simulink library "BlockLib"  (R2014b)
settings: Solver=ode45  StartTime=0.0  StopTime=10.0  RelTol=1e-3
libraries: BlockLib x3, dspsrcs4 x1
settings Model: Creator=kunalmenda  LastModifiedBy=kunalmenda

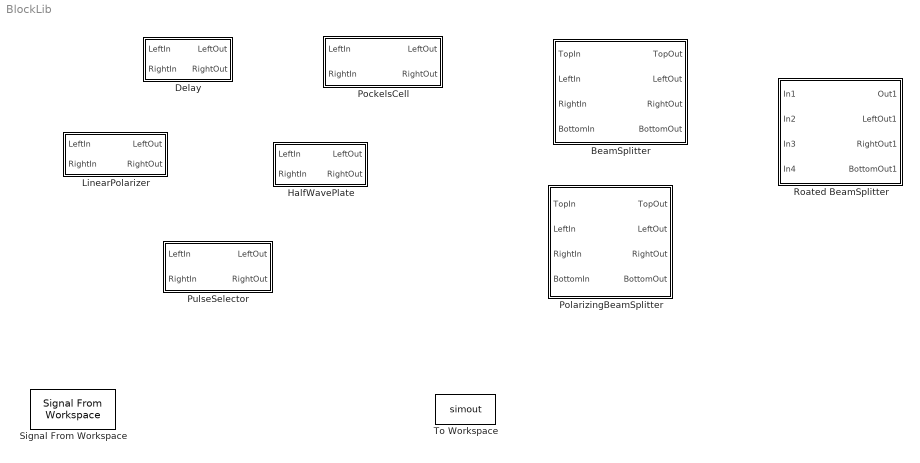
== system BlockLib ==
  BeamSplitter : Subsystem  mask{Transmittance=0.50, Reflectance=0.50, Ghost=0.01, BackReflectance=0.001}
      mask prompts: BackReflectance "Back Reflectance"
      mask TypeOptions Transmittance: BeamSplitter/Transmittance
      mask TypeOptions Reflectance: BeamSplitter/Reflectance
      mask TypeOptions Ghost: BeamSplitter/Ghost
      mask TypeOptions BackReflectance: BeamSplitter/BackReflectance
      mask Display:
      | image('BeamSplitter.jpg')
      | 
      | port_label('input',1,'TopIn');
      | port_label('input',2,'LeftIn');
      | port_label('input',3,'RightIn');
      | port_label('input',4,'BottomIn');
      | port_label('output',1,'TopOut');
      | port_label('output',2,'LeftOut');
      | port_label('output',3,'RightOut');
      | port_label('output',4,'BottomOut');
  Delay : Subsystem  mask{DelayAmt=10e-9}
      mask prompts: DelayAmt "Delay Amout"
      mask TypeOptions DelayAmt: Delay/DelayAmt
  HalfWavePlate : Subsystem  mask{Psi=pi/4, Transmittence=1}
      mask TypeOptions Psi: HalfWavePlate/Psi
      mask TypeOptions Transmittence: HalfWavePlate/Transmittence
  LinearPolarizer : Subsystem  mask{Psi=pi/4, Transmittence=0.81, ExtinctionRatio=200000000}
      mask TypeOptions Psi: LinearPolarizer/Psi
      mask TypeOptions Transmittence: LinearPolarizer/Transmittence
      mask TypeOptions ExtinctionRatio: LinearPolarizer/ExtinctionRatio
  PockelsCell : Subsystem  mask{PCTimings=[-1,1,38,40,103,105,168,170,220,274]*1e-9, ControlPowers=[0.5000, 1.0000,1.0000, 1.0000, 0.5000], Psi=pi/4}
      mask prompts: PCTimings "PC Timings"; ControlPowers "Control Powers"
      mask TypeOptions PCTimings: PockelsCell/PCTimings
      mask TypeOptions ControlPowers: PockelsCell/ControlPowers
      mask TypeOptions Psi: PockelsCell/Psi
  PolarizingBeamSplitter : Subsystem  mask{Psi=pi/2, Transmittance=0.50, Reflectance=0.50, Ghost=0.01, BackReflectance=0.001}
      mask prompts: BackReflectance "Back Reflectance"
      mask TypeOptions Psi: PolarizingBeamSplitter/Psi
      mask TypeOptions Transmittance: PolarizingBeamSplitter/Transmittance
      mask TypeOptions Reflectance: PolarizingBeamSplitter/Reflectance
      mask TypeOptions Ghost: PolarizingBeamSplitter/Ghost
      mask TypeOptions BackReflectance: PolarizingBeamSplitter/BackReflectance
      mask Display:
      | image('PolBeamSplitter.jpg')
      | 
      | port_label('input',1,'TopIn');
      | port_label('input',2,'LeftIn');
      | port_label('input',3,'RightIn');
      | port_label('input',4,'BottomIn');
      | port_label('output',1,'TopOut');
      | port_label('output',2,'LeftOut');
      | port_label('output',3,'RightOut');
      | port_label('output',4,'BottomOut');
  PulseSelector : Subsystem  mask{PCTimings=[-1,1,38,40,103,105,168,170,220,274]*1e-9, ControlPowers=[0.5000, 1.0000,1.0000, 1.0000, 0.5000]}
      mask prompts: PCTimings "PC Timings"; ControlPowers "Control Powers"
      mask TypeOptions PCTimings: PockelsCell/PCTimings
      mask TypeOptions ControlPowers: PockelsCell/ControlPowers
  Roated BeamSplitter : Subsystem  mask{Transmittance=0, Reflectance=0, Ghost=0, BackReflectance=0}
      mask TypeOptions Transmittance:
      | Level-2 MATLAB
      | S-Function/Transmittance
      mask TypeOptions Reflectance:
      | Level-2 MATLAB
      | S-Function/Reflectance
      mask TypeOptions Ghost:
      | Level-2 MATLAB
      | S-Function/Ghost
      mask TypeOptions BackReflectance:
      | Level-2 MATLAB
      | S-Function/BackReflectance
      mask Display:
      | image('BeamSplitterRot.jpeg')
      | 
      | port_label('input',1,'TopIn');
      | port_label('input',2,'LeftIn');
      | port_label('input',3,'RightIn');
      | port_label('input',4,'BottomIn');
      | port_label('output',1,'TopOut');
      | port_label('output',2,'LeftOut');
      | port_label('output',3,'RightOut');
      | port_label('output',4,'BottomOut');
  Signal From Workspace : dspsrcs4/Signal From Workspace  X=inputsignal  Ts=1  nsamps=1  OutputAfterFinalValue=Setting to zero  ignoreOrWarnInputAndFrameLengths=off
  To Workspace : ToWorkspace  VariableName=simout  SaveFormat=Timeseries  SampleTime=-1

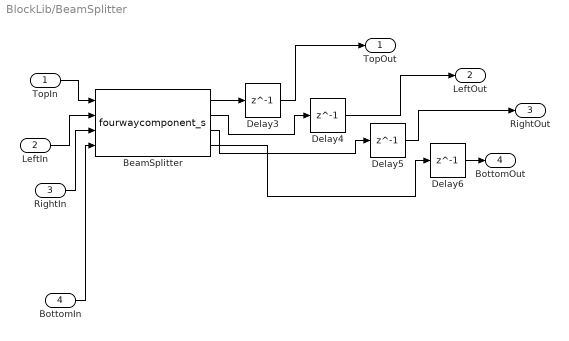
== system BlockLib/BeamSplitter ==
  TopIn : Inport
  LeftIn : Inport  Port=2
  RightIn : Inport  Port=3
  BottomIn : Inport  Port=4
  BeamSplitter : M-S-Function  FunctionName=fourwaycomponent_s  Parameters='BeamSplitter',Params  mask{Transmittance=Transmittance, Reflectance=Reflectance, Ghost=Ghost, BackReflectance=BackReflectance}
      mask prompts: BackReflectance "Back Reflectance"
      mask init:
      | Params.Transmittance = Transmittance;
      | Params.Reflectance = Reflectance;
      | Params.Ghost = Ghost;
      | Params.BackReflectance = BackReflectance;
      mask Display:
      | port_label('input',1,'TopIn');
      | port_label('input',2,'LeftIn');
      | port_label('input',3,'RightIn');
      | port_label('input',4,'BottomIn');
      | port_label('output',1,'TopOut');
      | port_label('output',2,'LeftOut');
      | port_label('output',3,'RightOut');
      | port_label('output',4,'BottomOut');
  Delay{3..6} (4 alike) : Delay  DelayLength=1  InitialCondition=0
  TopOut : Outport
  LeftOut : Outport  Port=2
  RightOut : Outport  Port=3
  BottomOut : Outport  Port=4
  wires:
  BeamSplitter/2 -> Delay4/1
  RightIn/1 -> BeamSplitter/3
  LeftIn/1 -> BeamSplitter/2
  Delay3/1 -> TopOut/1
  Delay4/1 -> LeftOut/1
  Delay6/1 -> BottomOut/1
  TopIn/1 -> BeamSplitter/1
  BottomIn/1 -> BeamSplitter/4
  BeamSplitter/1 -> Delay3/1
  BeamSplitter/3 -> Delay5/1
  Delay5/1 -> RightOut/1
  BeamSplitter/4 -> Delay6/1

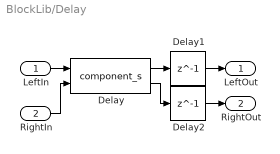
== system BlockLib/Delay ==
  LeftIn : Inport
  RightIn : Inport  Port=2
  Delay : M-S-Function  FunctionName=component_s  Parameters='Delay',Params  mask{DelayAmt=DelayAmt}
      mask prompts: DelayAmt "Delay Amout"
      mask init:
      | Params.DelayAmt = DelayAmt;
      mask Display:
      | port_label('input',1,'LeftIn');
      | port_label('input',2,'RightIn');
      | port_label('output',1,'LeftOut');
      | port_label('output',2,'RightOut');
  Delay1 : Delay  DelayLength=1  InitialCondition=0
  Delay2 : Delay  DelayLength=1  InitialCondition=0
  LeftOut : Outport
  RightOut : Outport  Port=2
  wires:
  Delay/1 -> Delay1/1
  Delay/2 -> Delay2/1
  LeftIn/1 -> Delay/1
  RightIn/1 -> Delay/2
  Delay1/1 -> LeftOut/1
  Delay2/1 -> RightOut/1

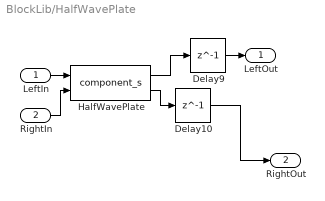
== system BlockLib/HalfWavePlate ==
  LeftIn : Inport
  RightIn : Inport  Port=2
  Delay10 : Delay  DelayLength=1  InitialCondition=0
  Delay9 : Delay  DelayLength=1  InitialCondition=0
  HalfWavePlate : M-S-Function  FunctionName=component_s  Parameters='HalfWavePlate',Params  mask{Psi=Psi, Transmittence=Transmittence}
      mask init:
      | Params.Psi = Psi;
      | Params.Transmittence = Transmittence;
      mask Display:
      | port_label('input',1,'LeftIn');
      | port_label('input',2,'RightIn');
      | port_label('output',1,'LeftOut');
      | port_label('output',2,'RightOut');
  LeftOut : Outport
  RightOut : Outport  Port=2
  wires:
  HalfWavePlate/1 -> Delay9/1
  Delay9/1 -> LeftOut/1
  LeftIn/1 -> HalfWavePlate/1
  RightIn/1 -> HalfWavePlate/2
  HalfWavePlate/2 -> Delay10/1
  Delay10/1 -> RightOut/1

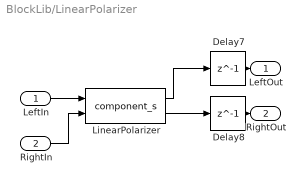
== system BlockLib/LinearPolarizer ==
  LeftIn : Inport
  RightIn : Inport  Port=2
  Delay7 : Delay  DelayLength=1  InitialCondition=0
  Delay8 : Delay  DelayLength=1  InitialCondition=0
  LinearPolarizer : M-S-Function  FunctionName=component_s  Parameters='LinearPolarizer',Params  mask{Psi=Psi, Transmittence=Transmittence, ExtinctionRatio=ExtinctionRatio}
      mask init:
      | Params.Psi = Psi;
      | Params.Transmittence = Transmittence;
      | Params.ExtinctionRatio = ExtinctionRatio;
      mask Display:
      | port_label('input',1,'LeftIn');
      | port_label('input',2,'RightIn');
      | port_label('output',1,'LeftOut');
      | port_label('output',2,'RightOut');
  LeftOut : Outport
  RightOut : Outport  Port=2
  wires:
  Delay8/1 -> RightOut/1
  RightIn/1 -> LinearPolarizer/2
  Delay7/1 -> LeftOut/1
  LeftIn/1 -> LinearPolarizer/1
  LinearPolarizer/1 -> Delay7/1
  LinearPolarizer/2 -> Delay8/1

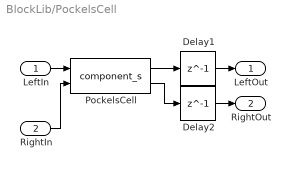
== system BlockLib/PockelsCell ==
  LeftIn : Inport
  RightIn : Inport  Port=2
  Delay1 : Delay  DelayLength=1  InitialCondition=0
  Delay2 : Delay  DelayLength=1  InitialCondition=0
  PockelsCell : M-S-Function  FunctionName=component_s  Parameters='PockelsCell',Params  mask{PCTimings=PCTimings, ControlPowers=ControlPowers, Psi=Psi}
      mask prompts: PCTimings "PC Timings"; ControlPowers "Control Powers"
      mask init:
      | Params.PCTimings = PCTimings;
      | Params.ControlPowers = ControlPowers;
      | Params.Psi = Psi;
      mask Display:
      | port_label('input',1,'LeftIn');
      | port_label('input',2,'RightIn');
      | port_label('output',1,'LeftOut');
      | port_label('output',2,'RightOut');
  LeftOut : Outport
  RightOut : Outport  Port=2
  wires:
  RightIn/1 -> PockelsCell/2
  PockelsCell/1 -> Delay1/1
  LeftIn/1 -> PockelsCell/1
  PockelsCell/2 -> Delay2/1
  Delay2/1 -> RightOut/1
  Delay1/1 -> LeftOut/1

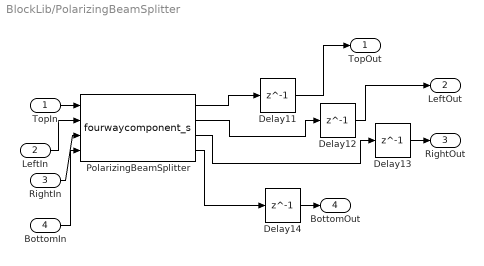
== system BlockLib/PolarizingBeamSplitter ==
  TopIn : Inport
  LeftIn : Inport  Port=2
  RightIn : Inport  Port=3
  BottomIn : Inport  Port=4
  Delay{11..14} (4 alike) : Delay  DelayLength=1  InitialCondition=0
  PolarizingBeamSplitter : M-S-Function  FunctionName=fourwaycomponent_s  Parameters='PolarizingBeamSplitter',Params  mask{Psi=Psi, Transmittance=Transmittance, Reflectance=Reflectance, Ghost=Ghost, BackReflectance=BackReflectance}
      mask prompts: BackReflectance "Back Reflectance"
      mask init:
      | Params.Psi = Psi;
      | Params.Transmittance = Transmittance;
      | Params.Reflectance = Reflectance;
      | Params.Ghost = Ghost;
      | Params.BackReflectance = BackReflectance;
      mask Display:
      | port_label('input',1,'TopIn');
      | port_label('input',2,'LeftIn');
      | port_label('input',3,'RightIn');
      | port_label('input',4,'BottomIn');
      | port_label('output',1,'TopOut');
      | port_label('output',2,'LeftOut');
      | port_label('output',3,'RightOut');
      | port_label('output',4,'BottomOut');
  TopOut : Outport
  LeftOut : Outport  Port=2
  RightOut : Outport  Port=3
  BottomOut : Outport  Port=4
  wires:
  RightIn/1 -> PolarizingBeamSplitter/3
  TopIn/1 -> PolarizingBeamSplitter/1
  Delay13/1 -> RightOut/1
  LeftIn/1 -> PolarizingBeamSplitter/2
  BottomIn/1 -> PolarizingBeamSplitter/4
  Delay11/1 -> TopOut/1
  Delay14/1 -> BottomOut/1
  Delay12/1 -> LeftOut/1
  PolarizingBeamSplitter/2 -> Delay12/1
  PolarizingBeamSplitter/1 -> Delay11/1
  PolarizingBeamSplitter/3 -> Delay13/1
  PolarizingBeamSplitter/4 -> Delay14/1

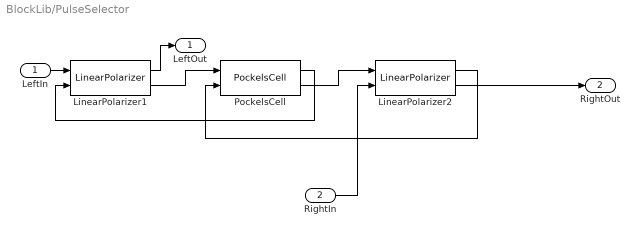
== system BlockLib/PulseSelector ==
  LeftIn : Inport
  RightIn : Inport  Port=2
  LinearPolarizer1 : BlockLib/LinearPolarizer  Psi=0  Transmittence=0.81  ExtinctionRatio=200000000
  LinearPolarizer2 : BlockLib/LinearPolarizer  Psi=pi/2  Transmittence=0.81  ExtinctionRatio=200000000
  PockelsCell : BlockLib/PockelsCell  PCTimings=PCTimings  ControlPowers=ControlPowers  Psi=pi/4
  LeftOut : Outport
  RightOut : Outport  Port=2
  wires:
  LeftIn/1 -> LinearPolarizer1/1
  LinearPolarizer1/2 -> PockelsCell/1
  PockelsCell/2 -> LinearPolarizer2/1
  RightIn/1 -> LinearPolarizer2/2
  LinearPolarizer2/1 -> PockelsCell/2
  PockelsCell/1 -> LinearPolarizer1/2
  LinearPolarizer1/1 -> LeftOut/1
  LinearPolarizer2/2 -> RightOut/1

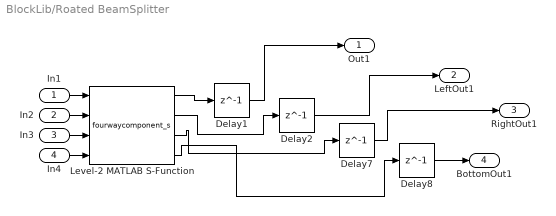
== system BlockLib/Roated BeamSplitter ==
  In1 : Inport
  In2 : Inport  Port=2
  In3 : Inport  Port=3
  In4 : Inport  Port=4
  Delay{1..2,7..8} (4 alike) : Delay  DelayLength=1  InitialCondition=0
  Level-2 MATLAB S-Function : M-S-Function  FunctionName=fourwaycomponent_s  Parameters='BeamSplitterRotated',Parameters  mask{Transmittance=Transmittance, Reflectance=Reflectance, Ghost=Ghost, BackReflectance=BackReflectance}
      mask init:
      | Parameters.Transmittance = Transmittance;
      | Parameters.Reflectance = Reflectance;
      | Parameters.Ghost = Ghost;
      | Parameters.BackReflectance = BackReflectance;
  Out1 : Outport
  LeftOut1 : Outport  Port=2
  RightOut1 : Outport  Port=3
  BottomOut1 : Outport  Port=4
  wires:
  Delay8/1 -> BottomOut1/1
  Delay2/1 -> LeftOut1/1
  In4/1 -> Level-2 MATLAB S-Function/4
  In3/1 -> Level-2 MATLAB S-Function/3
  In2/1 -> Level-2 MATLAB S-Function/2
  Level-2 MATLAB S-Function/1 -> Delay1/1
  Level-2 MATLAB S-Function/4 -> Delay8/1
  Delay7/1 -> RightOut1/1
  Delay1/1 -> Out1/1
  Level-2 MATLAB S-Function/2 -> Delay2/1
  In1/1 -> Level-2 MATLAB S-Function/1
  Level-2 MATLAB S-Function/3 -> Delay7/1
